simulink model "BuckyWagon_01"  (Simulink 7.5)
settings: Solver=FixedStepDiscrete  StartTime=0.0  StopTime=10.0  RelTol=1e-3
PreLoadFcn:
  | try, eval([bdroot '_setup']); catch, eval('model_setup', ''); end
InitFcn:
  | try, eval([bdroot '_setup']); catch, eval('model_setup', ''); end
undefined symbols (not defined in the file or in its folder): ECU565, High, Low, miniviewSetup, motohawk_build_version, motohawk_get_faults, motohawk_setup_toolchains, motohawk_trunc_name, motohawk_vardec_config_group, motohawk_vardec_path, tc, True
libraries: MotoHawk_lib x406, simulink x30, miniview_lib x10, motohawk_control_primitives_lib x9, MotoHawk_VDOGauge_lib x8, motohawk_engine_lib x7, motohawk_annotations_lib x2
(part 6 of 7)

== system BuckyWagon_01/Strategy/Sensors/Vehicle Speed ==
  Motor_Speed : Inport  OutDataType=sfix(16)  OutScaling=2^0
  Product : Product  OutDataType=sfix(16)  OutScaling=2^0  RndMeth=Zero
  motohawk_calibration : MotoHawk_lib/Calibration & Probing Blocks/motohawk_calibration  nam='OverallRatio'  val=0.002424  storage=Calibration  show_more=on  name_source=Use Parameter  data_type=Inherit from 'Default Value'  read_level=1  write_level=1  ovr_cals=on  view_as=Number  enum_struct={'Disabled', 'Enabled'}  vector_style=Wide Row  use_help_units=on  help='Used to calculate vehicle speed from motor speed'  units='mph/rpm'  use_header_enum=off  row_header_enum={}  col_header_enum={}  use_min_max=off  min_val=-inf  max_val=inf  use_precision=on  precision='1.4'  gain=1  offset=0  exp=1  use_mototune_group=on  mototune_group='Sensors | Vehicle Speed'
  motohawk_override_abs : MotoHawk_lib/Calibration & Probing Blocks/motohawk_override_abs  SystemSampleTime=-1  parent_name='Vehicle_Speed'  parent_val=0  show_more=off  name_source=Use Parameter  parent_read_level=1  parent_override_level=1  view_as=Number  enum_struct={'Disabled', 'Enabled'}  use_help_units=off  parent_help=''  parent_units=''  use_min_max=off  parent_min=-inf  parent_max=inf  use_precision=off  parent_precision=''  parent_gain=1  parent_offset=0  parent_exp=1  use_mototune_group=off  parent_group=motohawk_vardec_path(gcb)
  motohawk_probe : MotoHawk_lib/Calibration & Probing Blocks/motohawk_probe  nam='Vehicle_Speed'  show_more=on  name_source=Use Parameter  read_level=1  view_as=Number  enum_struct={'Disabled', 'Enabled'}  vector_style=Wide Row  use_help_units=off  help=''  units=''  use_header_enum=off  row_header_enum={}  col_header_enum={}  use_precision=on  precision='1.3'  gain=1  offset=0  exp=1  use_mototune_group=off  mototune_group=motohawk_vardec_path(gcb)
  Vehicle_Speed : Outport  OutDataType=sfix(16)  OutScaling=2^0
  wires:
  Motor_Speed/1 -> Product/1
  motohawk_calibration/1 -> Product/2
  Product/1 -> motohawk_override_abs/1
  motohawk_override_abs/1 -> Vehicle_Speed/1, motohawk_probe/1

== system BuckyWagon_01/Main Power Relay/Background/Delay/MotoHawk S-R Flip-Flop ==
  note: MotoHawk S-R Flip-Flop
  S : Inport  OutDataType=sfix(16)  OutScaling=2^0
  R : Inport  Port=2  OutDataType=sfix(16)  OutScaling=2^0
  Logical Operator : Logic  Operator=OR  OutDataTypeMode=boolean  OutDataTypeStr=boolean
  Logical Operator1 : Logic  Operator=NOT  OutDataTypeMode=boolean  OutDataTypeStr=boolean
  Logical Operator2 : Logic  OutDataTypeMode=boolean  OutDataTypeStr=boolean
  Logical Operator3 : Logic  Operator=NOT  OutDataTypeMode=boolean  OutDataTypeStr=boolean
  Signal Specification : SignalSpecification  DataType=boolean  OutDataType=sfix(16)  OutScaling=2^0  OutDataTypeStr=boolean
  Signal Specification1 : SignalSpecification  DataType=boolean  OutDataType=sfix(16)  OutScaling=2^0  OutDataTypeStr=boolean
  Unit Delay : UnitDelay  X0=ic_bool  SampleTime=-1
  Q : Outport
  !Q : Outport  Port=2
  wires:
  Logical Operator3/1 -> !Q/1
  R/1 -> Signal Specification/1
  S/1 -> Signal Specification1/1
  Signal Specification1/1 -> Logical Operator/2
  Signal Specification/1 -> Logical Operator1/1
  Logical Operator2/1 -> Q/1, Unit Delay/1, Logical Operator3/1
  Unit Delay/1 -> Logical Operator/1
  Logical Operator/1 -> Logical Operator2/1
  Logical Operator1/1 -> Logical Operator2/2

== system BuckyWagon_01/Strategy/Actuators/ReverseInd/Enabled Subsystem ==
  Period (Cnt) : Inport  OutDataType=sfix(16)  OutScaling=2^0
  Enable : EnablePort  StatesWhenEnabling=reset
  Constant : Constant  OutDataTypeMode=int16  OutDataType=sfix(16)  OutScaling=2^0  OutDataTypeStr=int16
  Gain : Gain  Gain=0.5  ParameterDataType=sfix(16)  ParameterScaling=2^0  OutDataType=sfix(16)  OutScaling=2^0  OutDataTypeStr=Inherit: Same as input
  Relational Operator : RelationalOperator  Operator=<=  LogicOutDataTypeMode=boolean  OutDataTypeStr=boolean
  Sum : Sum  Inputs=|+-  OutDataType=sfix(16)  OutScaling=2^0
  Switch : Switch  Criteria=u2 > Threshold
  Unit Delay : UnitDelay  SampleTime=-1
  Out : Outport  OutDataType=sfix(16)  OutScaling=2^0  InitialOutput=[0]
  wires:
  Relational Operator/1 -> Out/1
  Gain/1 -> Relational Operator/1
  Period (Cnt)/1 -> Gain/1, Switch/3
  Switch/1 -> Sum/1
  Sum/1 -> Relational Operator/2, Unit Delay/1
  Unit Delay/1 -> Switch/1, Switch/2
  Constant/1 -> Sum/2

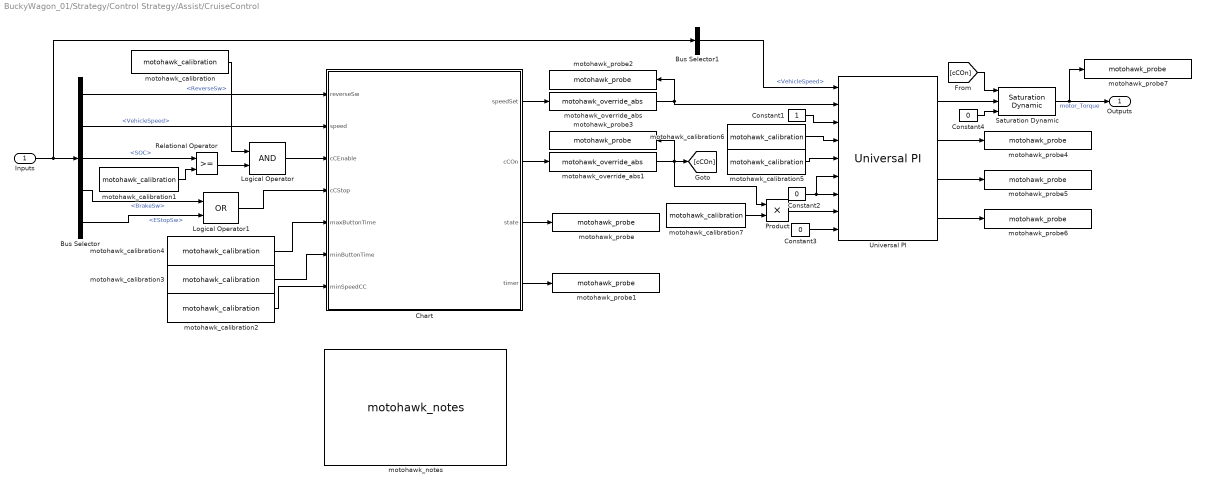
== system BuckyWagon_01/Strategy/Control Strategy/Assist/CruiseControl ==
  Inputs : Inport  OutDataType=sfix(16)  OutScaling=2^0
  Bus Selector : BusSelector  OutputSignals=ReverseSw,VehicleSpeed,SOC,BrakeSw,EStopSw
  Bus Selector1 : BusSelector  OutputSignals=VehicleSpeed
  Chart : Stateflow chart  TreatAsAtomicUnit=on
  Constant1 : Constant  OutDataType=sfix(16)  OutScaling=2^0
  Constant2 : Constant  Value=0  OutDataType=sfix(16)  OutScaling=2^0
  Constant3 : Constant  Value=0  OutDataType=sfix(16)  OutScaling=2^0
  Constant4 : Constant  Value=0  OutDataType=sfix(16)  OutScaling=2^0
  Logical Operator : Logic  IconShape=distinctive  AllPortsSameDT=off  OutDataTypeMode=boolean  OutDataTypeStr=boolean
  Logical Operator1 : Logic  Operator=OR  IconShape=distinctive  AllPortsSameDT=off  OutDataTypeMode=boolean  OutDataTypeStr=boolean
  Product : Product  OutDataType=sfix(16)  OutScaling=2^0  RndMeth=Zero
  Relational Operator : RelationalOperator  LogicOutDataTypeMode=boolean  OutDataTypeStr=boolean
  Saturation Dynamic : simulink/Discontinuities/Saturation Dynamic  SystemSampleTime=-1  OutMin=[]  OutMax=[]  OutDataTypeStr=Inherit: Same as second input  OutDataType=sfix(16)  OutScaling=2^-10  DoSatur=off
  Universal PI : motohawk_control_primitives_lib/Universal PI  Description=|  SystemSampleTime=-1  samp_time=-1
      | /* Name: ErrorGain Unit:mult ClassID:VAR StorageID:FLASH Access:RW4+RW3+NA2+NA1 TypeID:UINT4                   
      |    Gain:0.000000001 Min:0.000000000 Max:4.000000000 Format:10.9 UpdateID:REMOTE Help:"This gain is applied to "
      |    "the error term before it is used to calculate the P, I and D terms." VardecSig:6C */                       
      |                                                                                                                
      | /* Name: ITermLowerLim Unit:0 ClassID:VAR StorageID:FLASH Access:RW4+RW3+NA2+NA1 TypeID:SINT2 Gain:0.1         
      |    Min:-3276.8 Max:3276.7 Format:5.1 UpdateID:REMOTE Help:"Lower limit on the I-term value." VardecSig:6C */   
      |                                                                                                                
      | /* Name: ITermUpperLim ClassID:VAR StorageID:FLASH Access:RW4+RW3+NA2+NA1 TypeID:SINT2 Gain:0.1 Min:-3276.8    
      |    Max:3276.7 Format:5.1 UpdateID:REMOTE Help:"Upper limit on I-term value." VardecSig:6C */                   
      |                                                                                                                
      | /* Name: PIDOutLowerLim ClassID:VAR StorageID:FLASH Access:RW4+RW3+NA2+NA1 TypeID:SINT2 Gain:0.1               
      |    Min:-3276.8 Max:3276.7 Format:5.1 UpdateID:REMOTE Help:"Lower limit on PID output." VardecSig:6C */         
      |                                                                                                                
      | /* Name: PIDOutUpperLim ClassID:VAR StorageID:FLASH Access:RW4+RW3+NA2+NA1 TypeID:SINT2 Gain:0.1               
      |    Min:-3276.8 Max:3276.7 Format:3.1 UpdateID:REMOTE Help:"Upper limit on PID output." VardecSig:6C */
  motohawk_calibration : MotoHawk_lib/Calibration & Probing Blocks/motohawk_calibration  nam='cCEnable'  val=1  storage=Calibration  show_more=on  name_source=Use Parameter  data_type=uint8  read_level=1  write_level=1  ovr_cals=on  view_as=Enumeration  enum_struct={'Disabled', 'Enabled'}  vector_style=Wide Row  use_help_units=on  help='Enable Cruise Control.'  units=''  use_header_enum=off  row_header_enum={}  col_header_enum={}  use_min_max=off  min_val=-inf  max_val=inf  use_precision=off  precision=''  gain=1  offset=0  exp=1  use_mototune_group=off  mototune_group=motohawk_vardec_path(gcb)
  motohawk_calibration1 : MotoHawk_lib/Calibration & Probing Blocks/motohawk_calibration  nam='cCMinSOC'  val=0.02  storage=Calibration  show_more=on  name_source=Use Parameter  data_type=Inherit from 'Default Value'  read_level=1  write_level=1  ovr_cals=on  view_as=Number  enum_struct={'Disabled', 'Enabled'}  vector_style=Wide Row  use_help_units=on  help='Minimum SOC for cruise control to work.'  units='%'  use_header_enum=off  row_header_enum={}  col_header_enum={}  use_min_max=on  min_val=0  max_val=1  use_precision=on  precision='1.2'  gain=1  offset=0  exp=1  use_mototune_group=off  mototune_group=motohawk_vardec_path(gcb)
  motohawk_calibration2 : MotoHawk_lib/Calibration & Probing Blocks/motohawk_calibration  nam='cCMinSpeed'  val=10  storage=Calibration  show_more=on  name_source=Use Parameter  data_type=Inherit from 'Default Value'  read_level=1  write_level=1  ovr_cals=on  view_as=Number  enum_struct={'Disabled', 'Enabled'}  vector_style=Wide Row  use_help_units=on  help='Minimum speed for cruise control to work.'  units='mph'  use_header_enum=off  row_header_enum={}  col_header_enum={}  use_min_max=on  min_val=0  max_val=100  use_precision=on  precision='2.1'  gain=1  offset=0  exp=1  use_mototune_group=off  mototune_group=motohawk_vardec_path(gcb)
  motohawk_calibration3 : MotoHawk_lib/Calibration & Probing Blocks/motohawk_calibration  nam='cCMinButtonTime'  val=2  storage=Calibration  show_more=on  name_source=Use Parameter  data_type=uint8  read_level=1  write_level=1  ovr_cals=on  view_as=Number  enum_struct={'Disabled', 'Enabled'}  vector_style=Wide Row  use_help_units=on  help='Minimum time for button press or unpress.'  units='s'  use_header_enum=off  row_header_enum={}  col_header_enum={}  use_min_max=on  min_val=0  max_val=255/0.005  use_precision=on  precision='1.3'  gain=0.005  offset=0  exp=1  use_mototune_group=off  mototune_group=motohawk_vardec_path(gcb)
  motohawk_calibration4 : MotoHawk_lib/Calibration & Probing Blocks/motohawk_calibration  nam='cCMaxButtonTime'  val=80  storage=Calibration  show_more=on  name_source=Use Parameter  data_type=uint8  read_level=1  write_level=1  ovr_cals=on  view_as=Number  enum_struct={'Disabled', 'Enabled'}  vector_style=Wide Row  use_help_units=on  help='Maximum time for button press or unpress.'  units='s'  use_header_enum=off  row_header_enum={}  col_header_enum={}  use_min_max=on  min_val=0  max_val=255/0.005  use_precision=on  precision='1.3'  gain=0.005  offset=0  exp=1  use_mototune_group=off  mototune_group=motohawk_vardec_path(gcb)
  motohawk_calibration5 : MotoHawk_lib/Calibration & Probing Blocks/motohawk_calibration  nam='cCk_I'  val=0.015  storage=Calibration  show_more=on  name_source=Use Parameter  data_type=Inherit from 'Default Value'  read_level=1  write_level=1  ovr_cals=on  view_as=Number  enum_struct={'Disabled', 'Enabled'}  vector_style=Wide Row  use_help_units=on  help='Integrator gain for cruise control PI.'  units=''  use_header_enum=off  row_header_enum={}  col_header_enum={}  use_min_max=on  min_val=0  max_val=1  use_precision=on  precision='1.4'  gain=1  offset=0  exp=1  use_mototune_group=off  mototune_group=motohawk_vardec_path(gcb)
  motohawk_calibration6 : MotoHawk_lib/Calibration & Probing Blocks/motohawk_calibration  nam='cCk_P'  val=0.125  storage=Calibration  show_more=on  name_source=Use Parameter  data_type=Inherit from 'Default Value'  read_level=1  write_level=1  ovr_cals=on  view_as=Number  enum_struct={'Disabled', 'Enabled'}  vector_style=Wide Row  use_help_units=on  help='Integrator gain for cruise control PI.'  units=''  use_header_enum=off  row_header_enum={}  col_header_enum={}  use_min_max=on  min_val=0  max_val=1  use_precision=on  precision='1.4'  gain=1  offset=0  exp=1  use_mototune_group=off  mototune_group=motohawk_vardec_path(gcb)
  motohawk_calibration7 : MotoHawk_lib/Calibration & Probing Blocks/motohawk_calibration  nam='cCk_MaxAccel'  val=0.5  storage=Calibration  show_more=on  name_source=Use Parameter  data_type=Inherit from 'Default Value'  read_level=1  write_level=1  ovr_cals=on  view_as=Number  enum_struct={'Disabled', 'Enabled'}  vector_style=Wide Row  use_help_units=on  help='Maximum Torque the cruise control can request.'  units='%'  use_header_enum=off  row_header_enum={}  col_header_enum={}  use_min_max=on  min_val=0  max_val=1  use_precision=on  precision='1.3'  gain=1  offset=0  exp=1  use_mototune_group=off  mototune_group=motohawk_vardec_path(gcb)
  motohawk_notes : motohawk_annotations_lib/motohawk_notes  BlockType_='Mototron_Notes'  desc=' \newline\fontsize{18}\bfCruise Control State\rm\fontsize{12}\newline\newline0 - Disabled\newline1 - Off\newline2 - PressOne\newline3 - WaitOne\newline4 - PressTwo\newline5 - On'  edit_text=' \newline\fontsize{18}\bfCruise Control State\rm\fontsize{12}\newline\newline0 - Disabled\newline1 - Off\newline2 - PressOne\newline3 - WaitOne\newline4 - PressTwo\newline5 - On'  edit_as=6
  motohawk_override_abs : MotoHawk_lib/Calibration & Probing Blocks/motohawk_override_abs  SystemSampleTime=-1  parent_name='cCSpeedSet'  parent_val=0  show_more=on  name_source=Use Parameter  parent_read_level=1  parent_override_level=1  view_as=Number  enum_struct={'Disabled', 'Enabled'}  use_help_units=off  parent_help=''  parent_units=''  use_min_max=off  parent_min=-inf  parent_max=inf  use_precision=on  parent_precision='1.1'  parent_gain=1  parent_offset=0  parent_exp=1  use_mototune_group=off  parent_group=motohawk_vardec_path(gcb)
  motohawk_override_abs1 : MotoHawk_lib/Calibration & Probing Blocks/motohawk_override_abs  SystemSampleTime=-1  parent_name='cCOn'  parent_val=0  show_more=on  name_source=Use Parameter  parent_read_level=1  parent_override_level=1  view_as=Number  enum_struct={'Disabled', 'Enabled'}  use_help_units=off  parent_help=''  parent_units=''  use_min_max=off  parent_min=-inf  parent_max=inf  use_precision=on  parent_precision='1.0'  parent_gain=1  parent_offset=0  parent_exp=1  use_mototune_group=off  parent_group=motohawk_vardec_path(gcb)
  motohawk_probe : MotoHawk_lib/Calibration & Probing Blocks/motohawk_probe  nam='cCState'  show_more=on  name_source=Use Parameter  read_level=1  view_as=Enumeration  enum_struct={'Disabled','Off','Press1','Wait1','Press2','On'}  vector_style=Wide Row  use_help_units=off  help=''  units=''  use_header_enum=off  row_header_enum={}  col_header_enum={}  use_precision=off  precision=''  gain=1  offset=0  exp=1  use_mototune_group=off  mototune_group=motohawk_vardec_path(gcb)
  motohawk_probe1 : MotoHawk_lib/Calibration & Probing Blocks/motohawk_probe  nam='cCTimer'  show_more=on  name_source=Use Parameter  read_level=1  view_as=Number  enum_struct={'Disabled','Off','Press1','Wait1','Press2','On'}  vector_style=Wide Row  use_help_units=off  help=''  units=''  use_header_enum=off  row_header_enum={}  col_header_enum={}  use_precision=on  precision='1.3'  gain=0.005  offset=0  exp=1  use_mototune_group=off  mototune_group=motohawk_vardec_path(gcb)
  motohawk_probe2 : MotoHawk_lib/Calibration & Probing Blocks/motohawk_probe  nam='cCSpeedSet'  show_more=on  name_source=Use Parameter  read_level=1  view_as=Number  enum_struct={'Disabled','Off','Press1','Wait1','Press2','On'}  vector_style=Wide Row  use_help_units=off  help=''  units=''  use_header_enum=off  row_header_enum={}  col_header_enum={}  use_precision=on  precision='1.1'  gain=1  offset=0  exp=1  use_mototune_group=off  mototune_group=motohawk_vardec_path(gcb)
  motohawk_probe3 : MotoHawk_lib/Calibration & Probing Blocks/motohawk_probe  nam='cCOn'  show_more=on  name_source=Use Parameter  read_level=1  view_as=Number  enum_struct={'Disabled','Off','Press1','Wait1','Press2','On'}  vector_style=Wide Row  use_help_units=off  help=''  units=''  use_header_enum=off  row_header_enum={}  col_header_enum={}  use_precision=on  precision='1.0'  gain=1  offset=0  exp=1  use_mototune_group=off  mototune_group=motohawk_vardec_path(gcb)
  motohawk_probe4 : MotoHawk_lib/Calibration & Probing Blocks/motohawk_probe  nam='cCError'  show_more=on  name_source=Use Parameter  read_level=1  view_as=Number  enum_struct={'Disabled','Off','Press1','Wait1','Press2','On'}  vector_style=Wide Row  use_help_units=off  help=''  units=''  use_header_enum=off  row_header_enum={}  col_header_enum={}  use_precision=on  precision='1.3'  gain=1  offset=0  exp=1  use_mototune_group=off  mototune_group=motohawk_vardec_path(gcb)
  motohawk_probe5 : MotoHawk_lib/Calibration & Probing Blocks/motohawk_probe  nam='cCP_Term'  show_more=on  name_source=Use Parameter  read_level=1  view_as=Number  enum_struct={'Disabled','Off','Press1','Wait1','Press2','On'}  vector_style=Wide Row  use_help_units=off  help=''  units=''  use_header_enum=off  row_header_enum={}  col_header_enum={}  use_precision=on  precision='1.3'  gain=1  offset=0  exp=1  use_mototune_group=off  mototune_group=motohawk_vardec_path(gcb)
  motohawk_probe6 : MotoHawk_lib/Calibration & Probing Blocks/motohawk_probe  nam='cCI_Term'  show_more=on  name_source=Use Parameter  read_level=1  view_as=Number  enum_struct={'Disabled','Off','Press1','Wait1','Press2','On'}  vector_style=Wide Row  use_help_units=off  help=''  units=''  use_header_enum=off  row_header_enum={}  col_header_enum={}  use_precision=on  precision='1.3'  gain=1  offset=0  exp=1  use_mototune_group=off  mototune_group=motohawk_vardec_path(gcb)
  motohawk_probe7 : MotoHawk_lib/Calibration & Probing Blocks/motohawk_probe  nam='cCTrqReq'  show_more=on  name_source=Use Parameter  read_level=1  view_as=Number  enum_struct={'Disabled','Off','Press1','Wait1','Press2','On'}  vector_style=Wide Row  use_help_units=off  help=''  units=''  use_header_enum=off  row_header_enum={}  col_header_enum={}  use_precision=on  precision='1.3'  gain=1  offset=0  exp=1  use_mototune_group=off  mototune_group=motohawk_vardec_path(gcb)
  Outputs : Outport  OutDataType=sfix(16)  OutScaling=2^0
  wires:
  Saturation Dynamic/1 -> Outputs/1, motohawk_probe7/1  "motor_Torque"
  Inputs/1 -> Bus Selector/1, Bus Selector1/1
  Bus Selector/1 -> Chart/1(reverseSw)  "<ReverseSw>"
  Bus Selector/2 -> Chart/2(speed)  "<VehicleSpeed>"
  motohawk_calibration1/1 -> Relational Operator/2
  motohawk_calibration2/1 -> Chart/7(minSpeedCC)
  Logical Operator/1 -> Chart/3(cCEnable)
  motohawk_calibration/1 -> Logical Operator/1
  Relational Operator/1 -> Logical Operator/2
  Bus Selector/3 -> Relational Operator/1  "<SOC>"
  Bus Selector/4 -> Logical Operator1/1  "<BrakeSw>"
  Bus Selector/5 -> Logical Operator1/2  "<EStopSw>"
  Logical Operator1/1 -> Chart/4(cCStop)
  motohawk_calibration4/1 -> Chart/5(maxButtonTime)
  motohawk_calibration3/1 -> Chart/6(minButtonTime)
  Chart/3(state) -> motohawk_probe/1
  Chart/4(timer) -> motohawk_probe1/1
  Chart/1(speedSet) -> motohawk_override_abs/1
  motohawk_override_abs/1 -> motohawk_probe2/1, Universal PI/2
  Chart/2(cCOn) -> motohawk_override_abs1/1
  motohawk_override_abs1/1 -> motohawk_probe3/1, Product/1, [cCOn]
  motohawk_calibration5/1 -> Universal PI/5
  motohawk_calibration6/1 -> Universal PI/4
  Constant1/1 -> Universal PI/3
  Constant2/1 -> Universal PI/6, Universal PI/7
  Constant3/1 -> Universal PI/9
  Product/1 -> Universal PI/8
  motohawk_calibration7/1 -> Product/2
  Universal PI/1 -> Saturation Dynamic/2
  Universal PI/2 -> motohawk_probe4/1
  Universal PI/3 -> motohawk_probe5/1
  Universal PI/4 -> motohawk_probe6/1
  Bus Selector1/1 -> Universal PI/1  "<VehicleSpeed>"
  Constant4/1 -> Saturation Dynamic/3
  [cCOn] -> Saturation Dynamic/1

== system BuckyWagon_01/Strategy/Control Strategy/Assist/StallTorqueFault ==
  Inputs : Inport  OutDataType=sfix(16)  OutScaling=2^0
  Torque : Inport  Port=2  OutDataType=sfix(16)  OutScaling=2^0
  Abs : Abs  OutDataType=sfix(16)  OutScaling=2^0
  Bus Selector : BusSelector  OutputSignals=Accel,VehicleSpeed
  Constant : Constant  OutDataType=sfix(16)  OutScaling=2^0
  Constant1 : Constant  Value=-1  OutDataType=sfix(16)  OutScaling=2^0
  Constant2 : Constant  Value=0  OutDataType=sfix(16)  OutScaling=2^0
  Constant3 : Constant  Value=0  OutDataType=sfix(16)  OutScaling=2^0
  Constant4 : Constant  Value=0  OutDataType=sfix(16)  OutScaling=2^0
  Hysterisis : Subsystem  AncestorBlock=motohawk_control_primitives_lib/Hysterisis
      mask Display:
      | patch([0 0 1 1], [0 0.075 0.075 0], [230/255 0/255 0/255])
      | patch([0 0 1 1], [0.025 0.05 0.05 0.025], [150/255 0/255 0/255])
      | patch([0 0 1 1], [0 0.025 0.025 0], [0/255 0/255 0/255])
      | 
      | disp('HYSTERISIS')
  Integrator : motohawk_control_primitives_lib/Integrator  SystemSampleTime=-1  samp_time=0.005
  Product : Product  OutDataType=sfix(16)  OutScaling=2^0  RndMeth=Zero
  Relational Operator : RelationalOperator  Operator=<=  LogicOutDataTypeMode=boolean  OutDataTypeStr=boolean
  Relational Operator2 : RelationalOperator  Operator=>  LogicOutDataTypeMode=boolean  OutDataTypeStr=boolean
  Sum : Sum  Inputs=-+|  OutDataType=sfix(16)  OutScaling=2^0
  Switch : Switch  Criteria=u2 ~= 0  OutDataType=sfix(16)  OutScaling=2^0
  Switch1 : Switch  Criteria=u2 ~= 0  OutDataType=sfix(16)  OutScaling=2^0
  motohawk_calibration : MotoHawk_lib/Calibration & Probing Blocks/motohawk_calibration  nam='StallSpd'  val=1  storage=Calibration  show_more=on  name_source=Use Parameter  data_type=Inherit from 'Default Value'  read_level=1  write_level=1  ovr_cals=on  view_as=Number  enum_struct={'Disabled', 'Enabled'}  vector_style=Wide Row  use_help_units=on  help='Below this vehicle speed is concidered locked rotor.'  units='mph'  use_header_enum=off  row_header_enum={}  col_header_enum={}  use_min_max=on  min_val=0  max_val=100  use_precision=off  precision=''  gain=1  offset=0  exp=1  use_mototune_group=off  mototune_group=motohawk_vardec_path(gcb)
  motohawk_calibration1 : MotoHawk_lib/Calibration & Probing Blocks/motohawk_calibration  nam='StallTrqThres'  val=3  storage=Calibration  show_more=on  name_source=Use Parameter  data_type=Inherit from 'Default Value'  read_level=1  write_level=1  ovr_cals=on  view_as=Number  enum_struct={'Disabled', 'Enabled'}  vector_style=Wide Row  use_help_units=on  help='% seconds of torque allowed while speed is below thres.'  units='% s'  use_header_enum=off  row_header_enum={}  col_header_enum={}  use_min_max=off  min_val=-inf  max_val=inf  use_precision=off  precision=''  gain=1  offset=0  exp=1  use_mototune_group=off  mototune_group=motohawk_vardec_path(gcb)
  motohawk_calibration2 : MotoHawk_lib/Calibration & Probing Blocks/motohawk_calibration  nam='AccelRstThres'  val=0.05  storage=Calibration  show_more=on  name_source=Use Parameter  data_type=Inherit from 'Default Value'  read_level=1  write_level=1  ovr_cals=on  view_as=Number  enum_struct={'Disabled', 'Enabled'}  vector_style=Wide Row  use_help_units=on  help='Below this accel position fault can reset.'  units='%'  use_header_enum=off  row_header_enum={}  col_header_enum={}  use_min_max=on  min_val=0  max_val=1  use_precision=on  precision='1.2'  gain=1  offset=0  exp=1  use_mototune_group=off  mototune_group=motohawk_vardec_path(gcb)
  motohawk_calibration3 : MotoHawk_lib/Calibration & Probing Blocks/motohawk_calibration  nam='AccelRstSpd'  val=2  storage=Calibration  show_more=on  name_source=Use Parameter  data_type=Inherit from 'Default Value'  read_level=1  write_level=1  ovr_cals=on  view_as=Number  enum_struct={'Disabled', 'Enabled'}  vector_style=Wide Row  use_help_units=on  help='%'  units='Rate at which fault is cleared when accel is below thres.'  use_header_enum=off  row_header_enum={}  col_header_enum={}  use_min_max=off  min_val=-inf  max_val=inf  use_precision=off  precision=''  gain=1  offset=0  exp=1  use_mototune_group=off  mototune_group=motohawk_vardec_path(gcb)
  motohawk_fault_def1 : MotoHawk_lib/Fault Management Blocks/motohawk_fault_def  nam='LockedRotor'  mode=Disabled  id=0  x=25  y=50  input_suspected=on  indeterminate=off  increment_xy=on  downsample_count=1  ovr_cals=on  ovr_actions=off  show_actions=on  action1_name='DisableDrive'  action1_cond=Active  action2_name=''  action2_cond=(None)  action3_name=''  action3_cond=(None)  action4_name=''  action4_cond=(None)
  motohawk_probe : MotoHawk_lib/Calibration & Probing Blocks/motohawk_probe  nam='IntStallTorque'  show_more=off  name_source=Use Parameter  read_level=1  view_as=Number  enum_struct={'Disabled', 'Enabled'}  vector_style=Wide Row  use_help_units=off  help=''  units=''  use_header_enum=off  row_header_enum={}  col_header_enum={}  use_precision=off  precision=''  gain=1  offset=0  exp=1  use_mototune_group=off  mototune_group=motohawk_vardec_path(gcb)
  wires:
  Inputs/1 -> Bus Selector/1
  Bus Selector/2 -> Abs/1  "<VehicleSpeed>"
  motohawk_calibration/1 -> Relational Operator/2
  Relational Operator/1 -> Switch/2
  Switch/1 -> Product/1
  Torque/1 -> Product/2
  Integrator/1 -> Hysterisis/3(Signal), motohawk_probe/1
  motohawk_calibration1/1 -> Integrator/5, Hysterisis/1(HiThresh)
  Constant/1 -> Switch/1
  Constant1/1 -> Switch/3
  motohawk_calibration2/1 -> Relational Operator2/1
  Bus Selector/1 -> Relational Operator2/2  "<Accel>"
  Relational Operator2/1 -> Switch1/2
  motohawk_calibration3/1 -> Switch1/1
  Constant2/1 -> Switch1/3
  Switch1/1 -> Sum/1
  Product/1 -> Sum/2
  Sum/1 -> Integrator/1
  Constant3/1 -> Integrator/2, Integrator/3, Integrator/4
  Constant4/1 -> Hysterisis/2(LowThresh)
  Hysterisis/1(Threshold) -> motohawk_fault_def1/1
  Abs/1 -> Relational Operator/1

== system BuckyWagon_01/Strategy/Control Strategy/HV Controller/Contacter Controller ==
  Battery OK : Inport  DataType=boolean  OutDataType=sfix(16)  OutScaling=2^0  OutDataTypeStr=boolean
  Shutdown Command : Inport  Port=2  DataType=boolean  OutDataType=sfix(16)  OutScaling=2^0  OutDataTypeStr=boolean
  Contactor Status : Inport  Port=3  DataType=boolean  OutDataType=sfix(16)  OutScaling=2^0  OutDataTypeStr=boolean
  Delay : Subsystem
  Logical Operator2 : Logic  AllPortsSameDT=off  OutDataTypeMode=boolean  OutDataTypeStr=boolean
  Logical Operator3 : Logic  Operator=NOT  AllPortsSameDT=off  OutDataTypeMode=boolean  OutDataTypeStr=boolean
  Logical Operator4 : Logic  Inputs=3  AllPortsSameDT=off  OutDataTypeMode=boolean  OutDataTypeStr=boolean
  Logical Operator5 : Logic  Operator=NOT  AllPortsSameDT=off  OutDataTypeMode=boolean  OutDataTypeStr=boolean
  Logical Operator6 : Logic  Operator=NOT  AllPortsSameDT=off  OutDataTypeMode=boolean  OutDataTypeStr=boolean
  Relational Operator : RelationalOperator  LogicOutDataTypeMode=boolean  OutDataTypeStr=boolean
  Relational Operator1 : RelationalOperator  LogicOutDataTypeMode=boolean  OutDataTypeStr=boolean
  Time Since Enabled (With Input)1 : motohawk_control_primitives_lib/Time Since Enabled (With Input)1  SystemSampleTime=-1  nam='Contactor_Disable_Timer'  samp_time=-1  init=0  upperlim=3600*24
  Time Since Enabled (With Input)3 : motohawk_control_primitives_lib/Time Since Enabled (With Input)1  SystemSampleTime=-1  nam='Solectria_Enable_timer'  samp_time=-1  init=0  upperlim=3600*24
  motohawk_calibration : MotoHawk_lib/Calibration & Probing Blocks/motohawk_calibration  nam='Contactor_Disable_Delay'  val=0.5  storage=Calibration  show_more=on  name_source=Use Parameter  data_type=Inherit from 'Default Value'  read_level=1  write_level=1  ovr_cals=on  view_as=Number  enum_struct={'Disabled', 'Enabled'}  vector_style=Wide Row  use_help_units=off  help=''  units=''  use_header_enum=off  row_header_enum={}  col_header_enum={}  use_min_max=on  min_val=0  max_val=10  use_precision=on  precision='1.2'  gain=1  offset=0  exp=1  use_mototune_group=on  mototune_group=motohawk_vardec_path(gcb)
  motohawk_calibration1 : MotoHawk_lib/Calibration & Probing Blocks/motohawk_calibration  nam='Load_Enable_Delay'  val=2  storage=Calibration  show_more=on  name_source=Use Parameter  data_type=Inherit from 'Default Value'  read_level=1  write_level=1  ovr_cals=on  view_as=Number  enum_struct={'Disabled', 'Enabled'}  vector_style=Wide Row  use_help_units=off  help=''  units=''  use_header_enum=off  row_header_enum={}  col_header_enum={}  use_min_max=on  min_val=0  max_val=10  use_precision=on  precision='1.2'  gain=1  offset=0  exp=1  use_mototune_group=on  mototune_group=motohawk_vardec_path(gcb)
  motohawk_data_write : MotoHawk_lib/Data Storage Blocks/motohawk_data_write  source=Lookup By Name  structure=Scalar  operation=Write entire data structure at once  sz_vec=-1  sz_row=3  sz_col=2  typ=boolean  nam='MPRD_KeepAlive'  checkNull=off  write_read_only=off  struct_inst_name='Struct1'  struct_name='MyStruct'
  Contactor_Enable : Outport  DataType=boolean  OutDataType=sfix(16)  OutScaling=2^0  OutDataTypeStr=boolean
  Load_Enable : Outport  Port=2  DataType=boolean  OutDataType=sfix(16)  OutScaling=2^0  OutDataTypeStr=boolean
  wires:
  Shutdown Command/1 -> Time Since Enabled (With Input)1/1, Logical Operator3/1, Logical Operator5/1
  Time Since Enabled (With Input)1/1 -> Relational Operator/1
  Logical Operator2/1 -> Contactor_Enable/1, Delay/1(In)
  Logical Operator3/1 -> Logical Operator4/1
  Time Since Enabled (With Input)3/1 -> Relational Operator1/1
  Relational Operator1/1 -> Logical Operator4/2
  Logical Operator5/1 -> Time Since Enabled (With Input)3/1
  Logical Operator4/1 -> Load_Enable/1
  motohawk_calibration/1 -> Relational Operator/2
  motohawk_calibration1/1 -> Relational Operator1/2
  Relational Operator/1 -> Logical Operator6/1
  Logical Operator6/1 -> Logical Operator2/2
  Battery OK/1 -> Logical Operator2/1
  Delay/1(Out) -> motohawk_data_write/1
  Contactor Status/1 -> Logical Operator4/3

== system BuckyWagon_01/Strategy/Control Strategy/Regen/SOC_RampOut ==
  Torque_In : Inport  OutDataType=sfix(16)  OutScaling=2^0
  SOC : Inport  Port=2  OutDataType=sfix(16)  OutScaling=2^0
  Constant : Constant  OutDataType=sfix(16)  OutScaling=2^0
  Divide : Product  Inputs=*/  OutDataType=sfix(16)  OutScaling=2^-10
  Product : Product  OutDataType=sfix(16)  OutScaling=2^0  RndMeth=Zero
  Relational Operator : RelationalOperator  Operator=<=  LogicOutDataTypeMode=boolean  OutDataTypeStr=boolean
  Saturation : Saturate  UpperLimit=1  LowerLimit=0
  Sum : Sum  Inputs=-++  OutDataType=sfix(16)  OutScaling=2^0
  Switch : Switch  Criteria=u2 ~= 0
  motohawk_calibration : MotoHawk_lib/Calibration & Probing Blocks/motohawk_calibration  nam='RegenSOCRampWidth'  val=0.1  storage=Calibration  show_more=on  name_source=Use Parameter  data_type=Inherit from 'Default Value'  read_level=1  write_level=1  ovr_cals=on  view_as=Number  enum_struct={'Disabled', 'Enabled'}  vector_style=Wide Row  use_help_units=on  help='Regen ramps out this fast over max SOC'  units='%'  use_header_enum=off  row_header_enum={}  col_header_enum={}  use_min_max=on  min_val=0  max_val=1  use_precision=on  precision='1.3'  gain=1  offset=0  exp=1  use_mototune_group=off  mototune_group=motohawk_vardec_path(gcb)
  motohawk_calibration1 : MotoHawk_lib/Calibration & Probing Blocks/motohawk_calibration  nam='RegenMaxSOC'  val=0.1  storage=Calibration  show_more=on  name_source=Use Parameter  data_type=Inherit from 'Default Value'  read_level=1  write_level=1  ovr_cals=on  view_as=Number  enum_struct={'Disabled', 'Enabled'}  vector_style=Wide Row  use_help_units=on  help='Max SOC to Regen At'  units='%'  use_header_enum=off  row_header_enum={}  col_header_enum={}  use_min_max=off  min_val=0  max_val=1  use_precision=on  precision='1.2'  gain=1  offset=0  exp=1  use_mototune_group=off  mototune_group=motohawk_vardec_path(gcb)
  Torque_Out : Outport  OutDataType=sfix(16)  OutScaling=2^0
  wires:
  Saturation/1 -> Product/2
  motohawk_calibration1/1 -> Relational Operator/2, Sum/2
  SOC/1 -> Relational Operator/1, Sum/1
  Sum/1 -> Divide/1
  motohawk_calibration/1 -> Sum/3, Divide/2
  Relational Operator/1 -> Switch/2
  Divide/1 -> Switch/3
  Constant/1 -> Switch/1
  Torque_In/1 -> Product/1
  Switch/1 -> Saturation/1
  Product/1 -> Torque_Out/1

== system BuckyWagon_01/Strategy/Control Strategy/Regen/speed_RampOut ==
  Torque_In : Inport  OutDataType=sfix(16)  OutScaling=2^0
  speed : Inport  Port=2  OutDataType=sfix(16)  OutScaling=2^0
  Constant : Constant  OutDataType=sfix(16)  OutScaling=2^0
  Divide : Product  Inputs=*/  OutDataType=sfix(16)  OutScaling=2^-10
  Product : Product  OutDataType=sfix(16)  OutScaling=2^0  RndMeth=Zero
  Relational Operator : RelationalOperator  Operator=>  LogicOutDataTypeMode=boolean  OutDataTypeStr=boolean
  Saturation : Saturate  UpperLimit=1  LowerLimit=0
  Sum : Sum  Inputs=+-  OutDataType=sfix(16)  OutScaling=2^0
  Sum1 : Sum  Inputs=-+  OutDataType=sfix(16)  OutScaling=2^0
  Switch : Switch  Criteria=u2 ~= 0
  motohawk_data_def : MotoHawk_lib/Data Storage Blocks/motohawk_data_def  nam='RegenSpdRampStop'  container_nam=''  data=0  typ=double  struct_nam='MyStruct'  storage=NonVolatile  outputRef=off  use_vardec=on  window=Calibration  read_level=1  write_level=1  ovr_cals=on  view_as=Number  enum_struct={'Disabled', 'Enabled'}  vector_style=Wide Row  use_help_units=on  help='Speed at which regen is ramped out'  units='mph'  use_header_enum=off  row_header_enum=''  col_header_enum=''  use_min_max=on  min_val=0  max_val=5000  use_precision=on  precision=''  gain=1  offset=0  exp=1  use_mototune_group=off  mototune_group=motohawk_vardec_path(gcb)  eval_name=RegenSpdRampStop  data_stores=motohawk_sfun_data_def_data_stores  struct_instances=motohawk_sfun_data_def_struct_instances  vardecs=motohawk_sfun_data_def_vardecs
  motohawk_data_def1 : MotoHawk_lib/Data Storage Blocks/motohawk_data_def  nam='RegenSpdRampStart'  container_nam=''  data=0  typ=double  struct_nam='MyStruct'  storage=NonVolatile  outputRef=off  use_vardec=on  window=Calibration  read_level=1  write_level=1  ovr_cals=on  view_as=Number  enum_struct={'Disabled', 'Enabled'}  vector_style=Wide Row  use_help_units=on  help='Speed at which regen starts to ramp out'  units='mph'  use_header_enum=off  row_header_enum=''  col_header_enum=''  use_min_max=on  min_val=0  max_val=5000  use_precision=off  precision=''  gain=1  offset=0  exp=1  use_mototune_group=off  mototune_group=motohawk_vardec_path(gcb)  eval_name=RegenSpdRampStart  data_stores=motohawk_sfun_data_def_data_stores  struct_instances=motohawk_sfun_data_def_struct_instances  vardecs=motohawk_sfun_data_def_vardecs
  motohawk_data_read : MotoHawk_lib/Data Storage Blocks/motohawk_data_read  source=Lookup By Name  structure=Scalar  operation=Read scalar from location by index  sz_vec=4  sz_row=2  sz_col=3  typ=double  nam='RegenSpdRampStop'  checkNull=on  struct_inst_name='Struct1'  struct_nam='MyStruct'
  motohawk_data_read1 : MotoHawk_lib/Data Storage Blocks/motohawk_data_read  source=Lookup By Name  structure=Scalar  operation=Read scalar from location by index  sz_vec=4  sz_row=2  sz_col=3  typ=double  nam='RegenSpdRampStart'  checkNull=on  struct_inst_name='Struct1'  struct_nam='MyStruct'
  Torque_Out : Outport  OutDataType=sfix(16)  OutScaling=2^0
  wires:
  Saturation/1 -> Product/2
  Product/1 -> Torque_Out/1
  Switch/1 -> Saturation/1
  Torque_In/1 -> Product/1
  Constant/1 -> Switch/1
  Divide/1 -> Switch/3
  Relational Operator/1 -> Switch/2
  Sum1/1 -> Divide/2
  Sum/1 -> Divide/1
  motohawk_data_read1/1 -> Relational Operator/2, Sum1/2
  motohawk_data_read/1 -> Sum1/1, Sum/2
  speed/1 -> Relational Operator/1, Sum/1

== system BuckyWagon_01/Strategy/MiniViewDisplay/Down Button/Subsystem ==
  Trigger : TriggerPort  TriggerType=function-call
  Read CAN Message : MotoHawk_lib/CAN Blocks/Read CAN Message  nam=['CAN_' num2str(miniview_CAN_channel)]  bus=-2  msg=miniview_button_down  queue=1  slot='miniview_button_down'  valid=off  stale=off  labelwires=on
  Signal Specification : SignalSpecification  DataType=boolean  OutDataType=sfix(16)  OutScaling=2^0  OutDataTypeStr=boolean
  Signal Specification1 : SignalSpecification  DataType=uint8  OutDataType=sfix(16)  OutScaling=2^0  OutDataTypeStr=uint8
  Out1 : Outport  OutDataType=sfix(16)  OutScaling=2^0
  Out2 : Outport  Port=2  OutDataType=sfix(16)  OutScaling=2^0
  wires:
  Signal Specification1/1 -> Out2/1  "down count"
  Signal Specification/1 -> Out1/1  "down asserted"
  Read CAN Message/2 -> Signal Specification1/1  "down count"
  Read CAN Message/1 -> Signal Specification/1  "down asserted"

== system BuckyWagon_01/Strategy/MiniViewDisplay/GetFaultName/Fault Iterator ==
  function : TriggerPort  TriggerType=function-call
  Unit Delay : UnitDelay  SampleTime=-1
  motohawk_fault_iterator : MotoHawk_lib/Fault Management Blocks/motohawk_fault_iterator  criteria=Active Faults  loop=on
  motohawk_fault_name : MotoHawk_lib/Fault Management Blocks/motohawk_fault_name  width=size(char(motohawk_get_faults),2)+1
  Name : Outport  OutDataType=sfix(16)  OutScaling=2^0
  valid : Outport  Port=2  OutDataType=sfix(16)  OutScaling=2^0
  wires:
  motohawk_fault_iterator/2 -> Unit Delay/1, motohawk_fault_name/1
  Unit Delay/1 -> motohawk_fault_iterator/1
  motohawk_fault_iterator/1 -> valid/1
  motohawk_fault_name/1 -> Name/1

== system BuckyWagon_01/Strategy/MiniViewDisplay/Menu Button/Subsystem ==
  Trigger : TriggerPort  TriggerType=function-call
  Read CAN Message : MotoHawk_lib/CAN Blocks/Read CAN Message  nam=['CAN_' num2str(miniview_CAN_channel)]  bus=-2  msg=miniview_button_menu  queue=1  slot='miniview_button_menu'  valid=off  stale=off  labelwires=on
  Signal Specification : SignalSpecification  DataType=boolean  OutDataType=sfix(16)  OutScaling=2^0  OutDataTypeStr=boolean
  Signal Specification1 : SignalSpecification  DataType=uint8  OutDataType=sfix(16)  OutScaling=2^0  OutDataTypeStr=uint8
  Out1 : Outport  OutDataType=sfix(16)  OutScaling=2^0
  Out2 : Outport  Port=2  OutDataType=sfix(16)  OutScaling=2^0
  wires:
  Read CAN Message/1 -> Signal Specification/1  "menu asserted"
  Read CAN Message/2 -> Signal Specification1/1  "menu count"
  Signal Specification/1 -> Out1/1  "menu asserted"
  Signal Specification1/1 -> Out2/1  "menu count"

== system BuckyWagon_01/Strategy/MiniViewDisplay/Send String_efficient/Subsystem ==
  string # : Inport  OutDataType=sfix(16)  OutScaling=2^0
  string : Inport  Port=2  OutDataType=sfix(16)  OutScaling=2^0
  Trigger : TriggerPort  TriggerType=function-call
  Demux3 : Demux  Outputs=[7 7 3 1]
  Function-Call Generator : simulink/Ports & Subsystems/Function-Call Generator  sample_time=-1  numberOfIterations=1
  Function-Call Subsystem : Subsystem  TreatAsAtomicUnit=on
  Function-Call Subsystem1 : Subsystem  TreatAsAtomicUnit=on
  Send Substring (page 0) : miniview_lib/Send Substring (page 0)  SystemSampleTime=-1  miniview_CAN_channel=miniview_CAN_channel
  Send Substring (page 1) : miniview_lib/Send Substring (page 1)  SystemSampleTime=-1  miniview_CAN_channel=miniview_CAN_channel
  Send Substring (page 2) : miniview_lib/Send Substring (page 2)  SystemSampleTime=-1  miniview_CAN_channel=miniview_CAN_channel
  Terminator : Terminator
  Terminator1 : Terminator
  wires:
  Demux3/3 -> Send Substring (page 2)/2
  Demux3/2 -> Send Substring (page 1)/2, Function-Call Subsystem1/1(In1)
  Demux3/1 -> Send Substring (page 0)/2, Function-Call Subsystem/1(In1)
  string/1 -> Demux3/1  "string"
  string #/1 -> Send Substring (page 1)/1, Send Substring (page 2)/1, Send Substring (page 0)/1  "string #"
  Function-Call Generator/1 -> Send Substring (page 0)/Trigger
  Send Substring (page 0)/1 -> Function-Call Subsystem/Trigger
  Function-Call Subsystem/1(Out) -> Send Substring (page 1)/Trigger
  Send Substring (page 1)/1 -> Function-Call Subsystem1/Trigger
  Function-Call Subsystem1/1(Out) -> Send Substring (page 2)/Trigger
  Demux3/4 -> Terminator/1
  Send Substring (page 2)/1 -> Terminator1/1

== system BuckyWagon_01/Strategy/MiniViewDisplay/Up Button/Subsystem ==
  Trigger : TriggerPort  TriggerType=function-call
  Read CAN Message : MotoHawk_lib/CAN Blocks/Read CAN Message  nam=['CAN_' num2str(miniview_CAN_channel)]  bus=-2  msg=miniview_button_up  queue=1  slot='miniview_button_up'  valid=off  stale=off  labelwires=on
  Signal Specification : SignalSpecification  DataType=boolean  OutDataType=sfix(16)  OutScaling=2^0  OutDataTypeStr=boolean
  Signal Specification1 : SignalSpecification  DataType=uint8  OutDataType=sfix(16)  OutScaling=2^0  OutDataTypeStr=uint8
  Up Asserted : Outport  OutDataType=sfix(16)  OutScaling=2^0
  Up Count : Outport  Port=2  OutDataType=sfix(16)  OutScaling=2^0
  wires:
  Signal Specification1/1 -> Up Count/1  "up count"
  Signal Specification/1 -> Up Asserted/1  "up asserted"
  Read CAN Message/2 -> Signal Specification1/1  "up count"
  Read CAN Message/1 -> Signal Specification/1  "up asserted"

== system BuckyWagon_01/Strategy/Sensors/Brusa Charger/PluggedInDetect ==
  MainsVolt : Inport  OutDataType=sfix(16)  OutScaling=2^0
  Thres : Inport  Port=2  OutDataType=sfix(16)  OutScaling=2^0
  Time : Inport  Port=3  OutDataType=sfix(16)  OutScaling=2^0
  Chart : Stateflow chart  TreatAsAtomicUnit=on
  Relational Operator : RelationalOperator  Operator=>  LogicOutDataTypeMode=boolean  OutDataTypeStr=boolean
  pluggedIn : Outport  OutDataType=sfix(16)  OutScaling=2^0
  wires:
  MainsVolt/1 -> Relational Operator/1
  Thres/1 -> Relational Operator/2
  Chart/1(pluggedIn) -> pluggedIn/1
  Relational Operator/1 -> Chart/2(mainsOn)
  Time/1 -> Chart/1(histTime)

== system BuckyWagon_01/Strategy/Sensors/Linear Sensor Characterization/If Action Subsystem ==
  In : Inport  OutDataType=sfix(16)  OutScaling=2^0
  Action Port : ActionPort  ActionType=then
  Out : Outport  OutDataType=sfix(16)  OutScaling=2^0
  wires:
  In/1 -> Out/1

== system BuckyWagon_01/Strategy/Sensors/Linear Sensor Characterization/If Action Subsystem1 ==
  In : Inport  OutDataType=sfix(16)  OutScaling=2^0
  Action Port : ActionPort  ActionType=elseif
  Out : Outport  OutDataType=sfix(16)  OutScaling=2^0
  wires:
  In/1 -> Out/1

== system BuckyWagon_01/Strategy/Sensors/Linear Sensor Characterization/If Action Subsystem2 ==
  In : Inport  OutDataType=sfix(16)  OutScaling=2^0
  Action Port : ActionPort  ActionType=else
  Out : Outport  OutDataType=sfix(16)  OutScaling=2^0
  wires:
  In/1 -> Out/1

== system BuckyWagon_01/Strategy/Control Strategy/Assist/StallTorqueFault/Hysterisis ==
  HiThresh : Inport  OutDataType=sfix(16)  OutScaling=2^0
  LowThresh : Inport  Port=2  OutDataType=sfix(16)  OutScaling=2^0
  Signal : Inport  Port=3  OutDataType=sfix(16)  OutScaling=2^0
  Hysteresis : Subsystem
  LT : RelationalOperator  ZeroCross=off  InputSameDT=on
  LT1 : RelationalOperator  Operator=<=  ZeroCross=off  InputSameDT=on
  Threshold : Outport  OutDataType=sfix(16)  OutScaling=2^0
  wires:
  LT/1 -> Hysteresis/1(Hi)  "AboveHiTarget"
  LT1/1 -> Hysteresis/2(Lo)  "BelowLoTarget"
  Hysteresis/1("Out (Lo=0, Hi=1)") -> Threshold/1
  HiThresh/1 -> LT/2
  LowThresh/1 -> LT1/2
  Signal/1 -> LT/1, LT1/1

== system BuckyWagon_01/Strategy/Control Strategy/HV Controller/Contacter Controller/Delay ==
  note: Delay the rising and falling of a boolean signal
  In : Inport  OutDataType=sfix(16)  OutScaling=2^0
  Constant1 : Constant  Value=0  OutDataType=sfix(16)  OutScaling=2^0  OutDataTypeStr=Inherit: Inherit via back propagation
  Constant3 : Constant  Value=0  OutDataType=sfix(16)  OutScaling=2^0  OutDataTypeStr=Inherit: Inherit via back propagation
  Data Type Conversion : DataTypeConversion  OutDataType=sfix(16)  OutScaling=2^0  RndMeth=Zero
  Data Type Conversion1 : DataTypeConversion  OutDataType=sfix(16)  OutScaling=2^0  RndMeth=Zero
  Logical Operator : Logic  Operator=NOT  OutDataTypeMode=boolean  OutDataTypeStr=boolean
  Logical Operator1 : Logic  OutDataTypeMode=boolean  OutDataTypeStr=boolean
  Logical Operator2 : Logic  OutDataTypeMode=boolean  OutDataTypeStr=boolean
  MotoHawk S-R Flip-Flop : Subsystem  mask(MotoHawk S-R Flip-Flop){ic_bool=false}
      mask prompts: ic_bool "Initial condition Q (boolean)"
      mask help:
      | When input S (set) is TRUE, output Q is TRUE (and latched until reset).
      | When input R (reset) is TRUE, output Q is FALSE (and latched until set).
      | If both inputs S and R are TRUE, output Q is FALSE (reset wins).
      mask Display:
      | patch([0 0 1 1], [0 0.075 0.075 0], [230/255 0/255 0/255])
      | patch([0 0 1 1], [0.025 0.05 0.05 0.025], [150/255 0/255 0/255])
      | patch([0 0 1 1], [0 0.025 0.025 0], [0/255 0/255 0/255])
  Relational Operator1 : RelationalOperator  LogicOutDataTypeMode=boolean  OutDataTypeStr=boolean  ZeroCross=off  InputSameDT=on
  Relational Operator2 : RelationalOperator  LogicOutDataTypeMode=boolean  OutDataTypeStr=boolean  ZeroCross=off  InputSameDT=on
  Sum : Sum  Inputs=++|  OutDataType=sfix(16)  OutScaling=2^0  RndMeth=Zero  SaturateOnIntegerOverflow=on  InputSameDT=on
  Sum1 : Sum  Inputs=++|  OutDataType=sfix(16)  OutScaling=2^0  RndMeth=Zero  SaturateOnIntegerOverflow=on  InputSameDT=on
  Switch : Switch  Criteria=u2 ~= 0  Threshold=1  RndMeth=Zero  ZeroCross=off  InputSameDT=on
  Switch1 : Switch  Criteria=u2 ~= 0  Threshold=1  RndMeth=Zero  ZeroCross=off  InputSameDT=on
  Terminator : Terminator
  Unit Delay : UnitDelay  SampleTime=-1
  Unit Delay1 : UnitDelay  SampleTime=-1
  off delay : Constant  Value=10  OutDataType=sfix(16)  OutScaling=2^0
  on delay : Constant  Value=0  OutDataType=sfix(16)  OutScaling=2^0
  Out : Outport  OutDataType=sfix(16)  OutScaling=2^0
  wires:
  Logical Operator1/1 -> MotoHawk S-R Flip-Flop/2(R)
  Logical Operator2/1 -> MotoHawk S-R Flip-Flop/1(S)
  Relational Operator1/1 -> Logical Operator2/2
  Relational Operator2/1 -> Logical Operator1/2
  MotoHawk S-R Flip-Flop/2(!Q) -> Terminator/1
  MotoHawk S-R Flip-Flop/1(Q) -> Out/1
  off delay/1 -> Relational Operator2/2
  Logical Operator/1 -> Logical Operator1/1, Switch1/2, Data Type Conversion1/1
  Data Type Conversion1/1 -> Sum1/2  "0 to 1"
  Sum1/1 -> Switch1/1  "0 to 65535 (saturate hi)"
  Constant3/1 -> Switch1/3
  Switch1/1 -> Relational Operator2/1, Unit Delay1/1  "0 to 65535"
  In/1 -> Logical Operator/1, Logical Operator2/1, Switch/2, Data Type Conversion/1
  Data Type Conversion/1 -> Sum/2  "0 to 1"
  Sum/1 -> Switch/1  "0 to 65535 (saturate hi)"
  Constant1/1 -> Switch/3
  Switch/1 -> Unit Delay/1, Relational Operator1/1  "0 to 65535"
  on delay/1 -> Relational Operator1/2
  Unit Delay1/1 -> Sum1/1  "0 to 65535"
  Unit Delay/1 -> Sum/1  "0 to 65535"

== system BuckyWagon_01/Strategy/MiniViewDisplay/Send String_efficient/Subsystem/Function-Call Subsystem ==
  In1 : Inport  OutDataType=sfix(16)  OutScaling=2^0
  function : TriggerPort  TriggerType=function-call
  Compare To Zero : simulink/Logic and Bit Operations/Compare To Zero  SystemSampleTime=-1  relop=~=  LogicOutDataTypeMode=uint8  ZeroCross=off
  Enabled Subsystem : Subsystem  TreatAsAtomicUnit=on
  Logical Operator : Logic  Inputs=1  AllPortsSameDT=off  OutDataTypeMode=boolean  OutDataTypeStr=boolean
  Out : Outport  OutDataType=sfix(16)  OutScaling=2^0
  wires:
  Compare To Zero/1 -> Logical Operator/1
  In1/1 -> Compare To Zero/1
  Logical Operator/1 -> Enabled Subsystem/Enable
  Enabled Subsystem/1(Out1) -> Out/1

== system BuckyWagon_01/Strategy/MiniViewDisplay/Send String_efficient/Subsystem/Function-Call Subsystem1 ==
  In1 : Inport  OutDataType=sfix(16)  OutScaling=2^0
  function : TriggerPort  TriggerType=function-call
  Compare To Zero : simulink/Logic and Bit Operations/Compare To Zero  SystemSampleTime=-1  relop=~=  LogicOutDataTypeMode=uint8  ZeroCross=off
  Enabled Subsystem : Subsystem  TreatAsAtomicUnit=on
  Logical Operator : Logic  Inputs=1  AllPortsSameDT=off  OutDataTypeMode=boolean  OutDataTypeStr=boolean
  Out : Outport  OutDataType=sfix(16)  OutScaling=2^0
  wires:
  Enabled Subsystem/1(Out1) -> Out/1
  Logical Operator/1 -> Enabled Subsystem/Enable
  In1/1 -> Compare To Zero/1
  Compare To Zero/1 -> Logical Operator/1

== system BuckyWagon_01/Strategy/Control Strategy/Assist/StallTorqueFault/Hysterisis/Hysteresis ==
  note: Hi & !Lo => Hi
      | Lo & !Hi => Lo
      | Otherwise, Hold
  Hi : Inport  OutDataType=sfix(16)  OutScaling=2^0
  Lo : Inport  Port=2  OutDataType=sfix(16)  OutScaling=2^0
  Combinatorial  Logic : CombinatorialLogic  TruthTable=[0 0;0 1;1 1;0 0]
  Demux : Demux  Outputs=2
  Mux : Mux  Inputs=2
  Switch1 : Switch  Threshold=0.5  SaturateOnIntegerOverflow=on  InputSameDT=on
  Unit Delay : UnitDelay  SampleTime=-1
  "Out (Lo=0, Hi=1)" : Outport  OutDataType=sfix(16)  OutScaling=2^0
  wires:
  Mux/1 -> Combinatorial  Logic/1
  Combinatorial  Logic/1 -> Demux/1
  Demux/1 -> Switch1/1
  Demux/2 -> Switch1/2
  Unit Delay/1 -> Switch1/3
  Switch1/1 -> Unit Delay/1, "Out (Lo=0, Hi=1)"/1
  Hi/1 -> Mux/1
  Lo/1 -> Mux/2
